simulink model "lev_sys"  (R2021b)
settings: Solver=VariableStepAuto  StartTime=0.0  StopTime=30  RelTol=1e-3
values from neighbouring files (symbols this model uses):
  g = s(1:n,n+1:n+nb)    [MagLev.m]    (also in MagLev4coils.m = 9.8)
  K = m*g*x1*x1/i/i    (= 0.00013716864)    [MagLev.m]    (also in MagLev4coils.m = m*g*z1*z1/i/i)
  L = 0.00392    [MagLev.m]    (also in MagLev4coils.m = 0.00388)
  m = 0.03    [MagLev.m]    (also in MagLev4coils.m = 0.01)
  R = 10.8    [MagLev.m]    (also in MagLev4coils.m = 4)
settings Model: Creator=ik76  LastModifiedBy=ik76
settings SolverCC: ZeroCrossAlgorithm=Adaptive
settings OptimizationCC: BlockReduction=off  BooleanDataType=off
settings DebuggingCC: SaveWithParameterizedLinksMsg=none  UnderspecifiedInitializationDetection=Classic  MergeDetectMultiDrivingBlocksExec=none  SignalResolutionControl=TryResolveAllWithWarning  IgnoredZcDiagnostic=none
settings HardwareCC: TargetUnknown=on
settings ModelReferenceCC: PropagateSignalLabelsOutOfModel=off

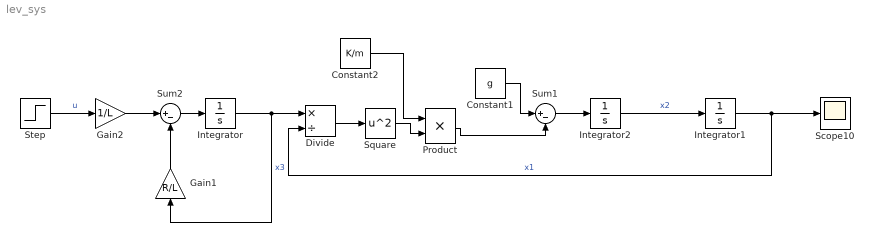
== system lev_sys ==
  Constant1 : Constant  Value=g
  Constant2 : Constant  Value=K/m
  Divide : Product  Inputs=*/
  Gain1 : Gain  Gain=R/L
  Gain2 : Gain  Gain=1/L
  Integrator : Integrator
  Integrator1 : Integrator  InitialCondition=-0.025
  Integrator2 : Integrator
  Product : Product
  Scope10 : Scope
  Square : Math  Operator=square  SaturateOnIntegerOverflow=on
  Step : Step  Time=0  After=2.5  SampleTime=0
  Sum1 : Sum  Inputs=|+-
  Sum2 : Sum  Inputs=|+-
  wires:
  Gain2/1 -> Sum2/1
  Gain1/1 -> Sum2/2
  Sum2/1 -> Integrator/1
  Integrator/1 -> Gain1/1, Divide/1  "x3"
  Divide/1 -> Square/1
  Square/1 -> Product/2
  Product/1 -> Sum1/2
  Sum1/1 -> Integrator2/1
  Constant2/1 -> Product/1
  Step/1 -> Gain2/1  "u"
  Integrator2/1 -> Integrator1/1  "x2"
  Constant1/1 -> Sum1/1
  Integrator1/1 -> Scope10/1, Divide/2  "x1"
